simulink model "Planar_PIDC"  (R2022b)
settings: Solver=VariableStepAuto  StartTime=0.0  StopTime=40  RelTol=1e-3
values from neighbouring files (symbols this model uses):
  I = [1; 1; 1; 0.5; 0.5]*0.2    [RobDyn4link.m]
  l = [1; 1; 1; 1; 2]*0.2    [RobDyn4link.m]
  lc = l./2    [RobDyn4link.m]
  m = [1; 1; 1; 0.3; 0.3]*1    [RobDyn4link.m]
  q0 = [pi/2; -pi/4; -1*pi/6;-pi/12;0;]    [RobDyn4link.m]
  theta_max = [0.915*pi; 0.915*pi; 0.915*pi; 0.915*pi; 0.915*pi;]    [RobDyn4link.m]
  theta_min = [-0.915*pi; -0.915*pi; -0.915*pi; -0.915*pi; -0.915*pi;]    [RobDyn4link.m]
undefined symbols (not defined in the file or in its folder): DiscIntNeverNeededParam
(part 2 of 3)

== matlab function Planar_PIDC/Subsystem6/Subsystem1/MATLAB Function ==
  data: theta input; C output; dtheta input; m input; l input; lc input
function C = fcn(theta,dtheta,m,l,lc)
theta1 = theta(1); theta2 = theta(2); theta3 = theta(3); theta4 = theta(4); theta5 = theta(5);
dtheta1 = dtheta(1); dtheta2 = dtheta(2); dtheta3 = dtheta(3); dtheta4 = dtheta(4); dtheta5 = dtheta(5);
% I1 = I(1); I2 = I(2); I3 = I(3); I4 = I(4); I5 = I(5);
m1 = m(1); m2 = m(2); m3 = m(3); m4 = m(4); m5 = m(5);
l1 = l(1); l2 = l(2); l3 = l(3); l4 = l(4); l5 = l(5);
lc1 = lc(1); lc2 = lc(2); lc3 = lc(3); lc4 = lc(4); lc5 = lc(5);

 
C =[- dtheta2*l1*l4*m5*sin(theta2 + theta3 + theta4) - dtheta3*l1*l4*m5*sin(theta2 + theta3 + theta4) - dtheta4*l1*l4*m5*sin(theta2 + theta3 + theta4) - dtheta2*l1*lc4*m4*sin(theta2 + theta3 + theta4) - dtheta3*l1*lc4*m4*sin(theta2 + theta3 + theta4) - dtheta4*l1*lc4*m4*sin(theta2 + theta3 + theta4) - dtheta3*l2*lc5*m5*sin(theta3 + theta4 + theta5) - dtheta4*l2*lc5*m5*sin(theta3 + theta4 + theta5) - dtheta5*l2*lc5*m5*sin(theta3 + theta4 + theta5) - dtheta2*l1*lc5*m5*sin(theta2 + theta3 + theta4 + theta5) - dtheta3*l1*lc5*m5*sin(theta2 + theta3 + theta4 + theta5) - dtheta4*l1*lc5*m5*sin(theta2 + theta3 + theta4 + theta5) - dtheta5*l1*lc5*m5*sin(theta2 + theta3 + theta4 + theta5) - dtheta2*l1*l3*m4*sin(theta2 + theta3) - dtheta2*l1*l3*m5*sin(theta2 + theta3) - dtheta3*l1*l3*m4*sin(theta2 + theta3) - dtheta3*l1*l3*m5*sin(theta2 + theta3) - dtheta3*l2*l4*m5*sin(theta3 + theta4) - dtheta4*l2*l4*m5*sin(theta3 + theta4) - dtheta2*l1*lc3*m3*sin(theta2 + theta3) - dtheta3*l1*lc3*m3*sin(theta2 + theta3) - dtheta3*l2*lc4*m4*sin(theta3 + theta4) - dtheta4*l2*lc4*m4*sin(theta3 + theta4) - dtheta4*l3*lc5*m5*sin(theta4 + theta5) - dtheta5*l3*lc5*m5*sin(theta4 + theta5) - dtheta2*l1*l2*m3*sin(theta2) - dtheta2*l1*l2*m4*sin(theta2) - dtheta2*l1*l2*m5*sin(theta2) - dtheta3*l2*l3*m4*sin(theta3) - dtheta3*l2*l3*m5*sin(theta3) - dtheta4*l3*l4*m5*sin(theta4) - dtheta2*l1*lc2*m2*sin(theta2) - dtheta3*l2*lc3*m3*sin(theta3) - dtheta4*l3*lc4*m4*sin(theta4) - dtheta5*l4*lc5*m5*sin(theta5), - dtheta1*l1*l4*m5*sin(theta2 + theta3 + theta4) - dtheta2*l1*l4*m5*sin(theta2 + theta3 + theta4) - dtheta3*l1*l4*m5*sin(theta2 + theta3 + theta4) - dtheta4*l1*l4*m5*sin(theta2 + theta3 + theta4) - dtheta1*l1*lc4*m4*sin(theta2 + theta3 + theta4) - dtheta2*l1*lc4*m4*sin(theta2 + theta3 + theta4) - dtheta3*l1*lc4*m4*sin(theta2 + theta3 + theta4) - dtheta4*l1*lc4*m4*sin(theta2 + theta3 + theta4) - dtheta3*l2*lc5*m5*sin(theta3 + theta4 + theta5) - dtheta4*l2*lc5*m5*sin(theta3 + theta4 + theta5) - dtheta5*l2*lc5*m5*sin(theta3 + theta4 + theta5) - dtheta1*l1*lc5*m5*sin(theta2 + theta3 + theta4 + theta5) - dtheta2*l1*lc5*m5*sin(theta2 + theta3 + theta4 + theta5) - dtheta3*l1*lc5*m5*sin(theta2 + theta3 + theta4 + theta5) - dtheta4*l1*lc5*m5*sin(theta2 + theta3 + theta4 + theta5) - dtheta5*l1*lc5*m5*sin(theta2 + theta3 + theta4 + theta5) - dtheta1*l1*l3*m4*sin(theta2 + theta3) - dtheta1*l1*l3*m5*sin(theta2 + theta3) - dtheta2*l1*l3*m4*sin(theta2 + theta3) - dtheta2*l1*l3*m5*sin(theta2 + theta3) - dtheta3*l1*l3*m4*sin(theta2 + theta3) - dtheta3*l1*l3*m5*sin(theta2 + theta3) - dtheta3*l2*l4*m5*sin(theta3 + theta4) - dtheta4*l2*l4*m5*sin(theta3 + theta4) - dtheta1*l1*lc3*m3*sin(theta2 + theta3) - dtheta2*l1*lc3*m3*sin(theta2 + theta3) - dtheta3*l1*lc3*m3*sin(theta2 + theta3) - dtheta3*l2*lc4*m4*sin(theta3 + theta4) - dtheta4*l2*lc4*m4*sin(theta3 + theta4) - dtheta4*l3*lc5*m5*sin(theta4 + theta5) - dtheta5*l3*lc5*m5*sin(theta4 + theta5) - dtheta1*l1*l2*m3*sin(theta2) - dtheta1*l1*l2*m4*sin(theta2) - dtheta2*l1*l2*m3*sin(theta2) - dtheta1*l1*l2*m5*sin(theta2) - dtheta2*l1*l2*m4*sin(theta2) - dtheta2*l1*l2*m5*sin(theta2) - dtheta3*l2*l3*m4*sin(theta3) - dtheta3*l2*l3*m5*sin(theta3) - dtheta4*l3*l4*m5*sin(theta4) - dtheta1*l1*lc2*m2*sin(theta2) - dtheta2*l1*lc2*m2*sin(theta2) - dtheta3*l2*lc3*m3*sin(theta3) - dtheta4*l3*lc4*m4*sin(theta4) - dtheta5*l4*lc5*m5*sin(theta5), - dtheta1*l1*l4*m5*sin(theta2 + theta3 + theta4) - dtheta2*l1*l4*m5*sin(theta2 + theta3 + theta4) - dtheta3*l1*l4*m5*sin(theta2 + theta3 + theta4) - dtheta4*l1*l4*m5*sin(theta2 + theta3 + theta4) - dtheta1*l1*lc4*m4*sin(theta2 + theta3 + theta4) - dtheta2*l1*lc4*m4*sin(theta2 + theta3 + theta4) - dtheta3*l1*lc4*m4*sin(theta2 + theta3 + theta4) - dtheta4*l1*lc4*m4*sin(theta2 + theta3 + theta4) - dtheta1*l2*lc5*m5*sin(theta3 + theta4 + theta5) - dtheta2*l2*lc5*m5*sin(theta3 + theta4 + theta5) - dtheta3*l2*lc5*m5*sin(theta3 + theta4 + theta5) - dtheta4*l2*lc5*m5*sin(theta3 + theta4 + theta5) - dtheta5*l2*lc5*m5*sin(theta3 + theta4 + theta5) - dtheta1*l1*lc5*m5*sin(theta2 + theta3 + theta4 + theta5) - dtheta2*l1*lc5*m5*sin(theta2 + theta3 + theta4 + theta5) - dtheta3*l1*lc5*m5*sin(theta2 + theta3 + theta4 + theta5) - dtheta4*l1*lc5*m5*sin(theta2 + theta3 + theta4 + theta5) - dtheta5*l1*lc5*m5*sin(theta2 + theta3 + theta4 + theta5) - dtheta1*l1*l3*m4*sin(theta2 + theta3) - dtheta1*l1*l3*m5*sin(theta2 + theta3) - dtheta2*l1*l3*m4*sin(theta2 + theta3) - dtheta2*l1*l3*m5*sin(theta2 + theta3) - dtheta3*l1*l3*m4*sin(theta2 + theta3) - dtheta3*l1*l3*m5*sin(theta2 + theta3) - dtheta1*l2*l4*m5*sin(theta3 + theta4) - dtheta2*l2*l4*m5*sin(theta3 + theta4) - dtheta3*l2*l4*m5*sin(theta3 + theta4) - dtheta4*l2*l4*m5*sin(theta3 + theta4) - dtheta1*l1*lc3*m3*sin(theta2 + theta3) - dtheta2*l1*lc3*m3*sin(theta2 + theta3) - dtheta3*l1*lc3*m3*sin(theta2 + theta3) - dtheta1*l2*lc4*m4*sin(theta3 + theta4) - dtheta2*l2*lc4*m4*sin(theta3 + theta4) - dtheta3*l2*lc4*m4*sin(theta3 + theta4) - dtheta4*l2*lc4*m4*sin(theta3 + theta4) - dtheta4*l3*lc5*m5*sin(theta4 + theta5) - dtheta5*l3*lc5*m5*sin(theta4 + theta5) - dtheta1*l2*l3*m4*sin(theta3) - dtheta1*l2*l3*m5*sin(theta3) - dtheta2*l2*l3*m4*sin(theta3) - dtheta2*l2*l3*m5*sin(theta3) - dtheta3*l2*l3*m4*sin(theta3) - dtheta3*l2*l3*m5*sin(theta3) - dtheta4*l3*l4*m5*sin(theta4) - dtheta1*l2*lc3*m3*sin(theta3) - dtheta2*l2*lc3*m3*sin(theta3) - dtheta3*l2*lc3*m3*sin(theta3) - dtheta4*l3*lc4*m4*sin(theta4) - dtheta5*l4*lc5*m5*sin(theta5), - dtheta1*l1*l4*m5*sin(theta2 + theta3 + theta4) - dtheta2*l1*l4*m5*sin(theta2 + theta3 + theta4) - dtheta3*l1*l4*m5*sin(theta2 + theta3 + theta4) - dtheta4*l1*l4*m5*sin(theta2 + theta3 + theta4) - dtheta1*l1*lc4*m4*sin(theta2 + theta3 + theta4) - dtheta2*l1*lc4*m4*sin(theta2 + theta3 + theta4) - dtheta3*l1*lc4*m4*sin(theta2 + theta3 + theta4) - dtheta4*l1*lc4*m4*sin(theta2 + theta3 + theta4) - dtheta1*l2*lc5*m5*sin(theta3 + theta4 + theta5) - dtheta2*l2*lc5*m5*sin(theta3 + theta4 + theta5) - dtheta3*l2*lc5*m5*sin(theta3 + theta4 + theta5) - dtheta4*l2*lc5*m5*sin(theta3 + theta4 + theta5) - dtheta5*l2*lc5*m5*sin(theta3 + theta4 + theta5) - dtheta1*l1*lc5*m5*sin(theta2 + theta3 + theta4 + theta5) - dtheta2*l1*lc5*m5*sin(theta2 + theta3 + theta4 + theta5) - dtheta3*l1*lc5*m5*sin(theta2 + theta3 + theta4 + theta5) - dtheta4*l1*lc5*m5*sin(theta2 + theta3 + theta4 + theta5) - dtheta5*l1*lc5*m5*sin(theta2 + theta3 + theta4 + theta5) - dtheta1*l2*l4*m5*sin(theta3 + theta4) - dtheta2*l2*l4*m5*sin(theta3 + theta4) - dtheta3*l2*l4*m5*sin(theta3 + theta4) - dtheta4*l2*l4*m5*sin(theta3 + theta4) - dtheta1*l2*lc4*m4*sin(theta3 + theta4) - dtheta2*l2*lc4*m4*sin(theta3 + theta4) - dtheta3*l2*lc4*m4*sin(theta3 + theta4) - dtheta4*l2*lc4*m4*sin(theta3 + theta4) - dtheta1*l3*lc5*m5*sin(theta4 + theta5) - dtheta2*l3*lc5*m5*sin(theta4 + theta5) - dtheta3*l3*lc5*m5*sin(theta4 + theta5) - dtheta4*l3*lc5*m5*sin(theta4 + theta5) - dtheta5*l3*lc5*m5*sin(theta4 + theta5) - dtheta1*l3*l4*m5*sin(theta4) - dtheta2*l3*l4*m5*sin(theta4) - dtheta3*l3*l4*m5*sin(theta4) - dtheta4*l3*l4*m5*sin(theta4) - dtheta1*l3*lc4*m4*sin(theta4) - dtheta2*l3*lc4*m4*sin(theta4) - dtheta3*l3*lc4*m4*sin(theta4) - dtheta4*l3*lc4*m4*sin(theta4) - dtheta5*l4*lc5*m5*sin(theta5), -lc5*m5*(l1*sin(theta2 + theta3 + theta4 + theta5) + l3*sin(theta4 + theta5) + l4*sin(theta5) + l2*sin(theta3 + theta4 + theta5))*(dtheta1 + dtheta2 + dtheta3 + dtheta4 + dtheta5);
                                                                                                                                                                                                                                                                                                                                                                                                                                                                                                                  dtheta1*l1*l4*m5*sin(theta2 + theta3 + theta4) + dtheta1*l1*lc4*m4*sin(theta2 + theta3 + theta4) - dtheta3*l2*lc5*m5*sin(theta3 + theta4 + theta5) - dtheta4*l2*lc5*m5*sin(theta3 + theta4 + theta5) - dtheta5*l2*lc5*m5*sin(theta3 + theta4 + theta5) + dtheta1*l1*lc5*m5*sin(theta2 + theta3 + theta4 + theta5) + dtheta1*l1*l3*m4*sin(theta2 + theta3) + dtheta1*l1*l3*m5*sin(theta2 + theta3) - dtheta3*l2*l4*m5*sin(theta3 + theta4) - dtheta4*l2*l4*m5*sin(theta3 + theta4) + dtheta1*l1*lc3*m3*sin(theta2 + theta3) - dtheta3*l2*lc4*m4*sin(theta3 + theta4) - dtheta4*l2*lc4*m4*sin(theta3 + theta4) - dtheta4*l3*lc5*m5*sin(theta4 + theta5) - dtheta5*l3*lc5*m5*sin(theta4 + theta5) + dtheta1*l1*l2*m3*sin(theta2) + dtheta1*l1*l2*m4*sin(theta2) + dtheta1*l1*l2*m5*sin(theta2) - dtheta3*l2*l3*m4*sin(theta3) - dtheta3*l2*l3*m5*sin(theta3) - dtheta4*l3*l4*m5*sin(theta4) + dtheta1*l1*lc2*m2*sin(theta2) - dtheta3*l2*lc3*m3*sin(theta3) - dtheta4*l3*lc4*m4*sin(theta4) - dtheta5*l4*lc5*m5*sin(theta5),                                                                                                                                                                                                                                                                                                                                                                                                                                                                                                                                                                                                                                                                                                                                                                                                                                                                                                                                                                                                                                                                                                                                                                                                                                                                                                                                                                                                                                                                                - dtheta4*(l2*l4*m5*sin(theta3 + theta4) + l2*lc4*m4*sin(theta3 + theta4) + l3*lc5*m5*sin(theta4 + theta5) + l3*l4*m5*sin(theta4) + l3*lc4*m4*sin(theta4) + l2*lc5*m5*sin(theta3 + theta4 + theta5)) - dtheta3*l2*(l3*m4*sin(theta3) + l3*m5*sin(theta3) + lc3*m3*sin(theta3) + lc5*m5*sin(theta3 + theta4 + theta5) + l4*m5*sin(theta3 + theta4) + lc4*m4*sin(theta3 + theta4)) - dtheta5*lc5*m5*(l3*sin(theta4 + theta5) + l4*sin(theta5) + l2*sin(theta3 + theta4 + theta5)),                                                                                                                                                                                                                                                                                                                                                                                                                                                                                                                                                                                                                                                                                                                                                                                                                                                                                                                                                                                                                                                                                               - dtheta1*l2*lc5*m5*sin(theta3 + theta4 + theta5) - dtheta2*l2*lc5*m5*sin(theta3 + theta4 + theta5) - dtheta3*l2*lc5*m5*sin(theta3 + theta4 + theta5) - dtheta4*l2*lc5*m5*sin(theta3 + theta4 + theta5) - dtheta5*l2*lc5*m5*sin(theta3 + theta4 + theta5) - dtheta1*l2*l4*m5*sin(theta3 + theta4) - dtheta2*l2*l4*m5*sin(theta3 + theta4) - dtheta3*l2*l4*m5*sin(theta3 + theta4) - dtheta4*l2*l4*m5*sin(theta3 + theta4) - dtheta1*l2*lc4*m4*sin(theta3 + theta4) - dtheta2*l2*lc4*m4*sin(theta3 + theta4) - dtheta3*l2*lc4*m4*sin(theta3 + theta4) - dtheta4*l2*lc4*m4*sin(theta3 + theta4) - dtheta4*l3*lc5*m5*sin(theta4 + theta5) - dtheta5*l3*lc5*m5*sin(theta4 + theta5) - dtheta1*l2*l3*m4*sin(theta3) - dtheta1*l2*l3*m5*sin(theta3) - dtheta2*l2*l3*m4*sin(theta3) - dtheta2*l2*l3*m5*sin(theta3) - dtheta3*l2*l3*m4*sin(theta3) - dtheta3*l2*l3*m5*sin(theta3) - dtheta4*l3*l4*m5*sin(theta4) - dtheta1*l2*lc3*m3*sin(theta3) - dtheta2*l2*lc3*m3*sin(theta3) - dtheta3*l2*lc3*m3*sin(theta3) - dtheta4*l3*lc4*m4*sin(theta4) - dtheta5*l4*lc5*m5*sin(theta5),                                                                                                                                                                                                                                                                                                                                                                                                                                                                                                                                                                                                                                                                                                                    - dtheta1*l2*lc5*m5*sin(theta3 + theta4 + theta5) - dtheta2*l2*lc5*m5*sin(theta3 + theta4 + theta5) - dtheta3*l2*lc5*m5*sin(theta3 + theta4 + theta5) - dtheta4*l2*lc5*m5*sin(theta3 + theta4 + theta5) - dtheta5*l2*lc5*m5*sin(theta3 + theta4 + theta5) - dtheta1*l2*l4*m5*sin(theta3 + theta4) - dtheta2*l2*l4*m5*sin(theta3 + theta4) - dtheta3*l2*l4*m5*sin(theta3 + theta4) - dtheta4*l2*l4*m5*sin(theta3 + theta4) - dtheta1*l2*lc4*m4*sin(theta3 + theta4) - dtheta2*l2*lc4*m4*sin(theta3 + theta4) - dtheta3*l2*lc4*m4*sin(theta3 + theta4) - dtheta4*l2*lc4*m4*sin(theta3 + theta4) - dtheta1*l3*lc5*m5*sin(theta4 + theta5) - dtheta2*l3*lc5*m5*sin(theta4 + theta5) - dtheta3*l3*lc5*m5*sin(theta4 + theta5) - dtheta4*l3*lc5*m5*sin(theta4 + theta5) - dtheta5*l3*lc5*m5*sin(theta4 + theta5) - dtheta1*l3*l4*m5*sin(theta4) - dtheta2*l3*l4*m5*sin(theta4) - dtheta3*l3*l4*m5*sin(theta4) - dtheta4*l3*l4*m5*sin(theta4) - dtheta1*l3*lc4*m4*sin(theta4) - dtheta2*l3*lc4*m4*sin(theta4) - dtheta3*l3*lc4*m4*sin(theta4) - dtheta4*l3*lc4*m4*sin(theta4) - dtheta5*l4*lc5*m5*sin(theta5),                                             -lc5*m5*(l3*sin(theta4 + theta5) + l4*sin(theta5) + l2*sin(theta3 + theta4 + theta5))*(dtheta1 + dtheta2 + dtheta3 + dtheta4 + dtheta5);
                                                                                                                                                                                                                                                                                                                                                                                                                                                                                                                                                                                                   dtheta1*l1*l4*m5*sin(theta2 + theta3 + theta4) + dtheta1*l1*lc4*m4*sin(theta2 + theta3 + theta4) + dtheta1*l2*lc5*m5*sin(theta3 + theta4 + theta5) + dtheta2*l2*lc5*m5*sin(theta3 + theta4 + theta5) + dtheta1*l1*lc5*m5*sin(theta2 + theta3 + theta4 + theta5) + dtheta1*l1*l3*m4*sin(theta2 + theta3) + dtheta1*l1*l3*m5*sin(theta2 + theta3) + dtheta1*l2*l4*m5*sin(theta3 + theta4) + dtheta2*l2*l4*m5*sin(theta3 + theta4) + dtheta1*l1*lc3*m3*sin(theta2 + theta3) + dtheta1*l2*lc4*m4*sin(theta3 + theta4) + dtheta2*l2*lc4*m4*sin(theta3 + theta4) - dtheta4*l3*lc5*m5*sin(theta4 + theta5) - dtheta5*l3*lc5*m5*sin(theta4 + theta5) + dtheta1*l2*l3*m4*sin(theta3) + dtheta1*l2*l3*m5*sin(theta3) + dtheta2*l2*l3*m4*sin(theta3) + dtheta2*l2*l3*m5*sin(theta3) - dtheta4*l3*l4*m5*sin(theta4) + dtheta1*l2*lc3*m3*sin(theta3) + dtheta2*l2*lc3*m3*sin(theta3) - dtheta4*l3*lc4*m4*sin(theta4) - dtheta5*l4*lc5*m5*sin(theta5),                                                                                                                                                                                                                                                                                                                                                                                                                                                                                                                                                                                                                                                                                                                                                                                                                                                                                                                                                                                                                                                                                                                                                                                                                                                                                                                                                                                                               dtheta1*(l2*l4*m5*sin(theta3 + theta4) + l2*lc4*m4*sin(theta3 + theta4) + l2*l3*m4*sin(theta3) + l2*l3*m5*sin(theta3) + l2*lc3*m3*sin(theta3) + l2*lc5*m5*sin(theta3 + theta4 + theta5)) - dtheta5*(l3*lc5*m5*sin(theta4 + theta5) + l4*lc5*m5*sin(theta5)) + dtheta2*(l2*l4*m5*sin(theta3 + theta4) + l2*lc4*m4*sin(theta3 + theta4) + l2*l3*m4*sin(theta3) + l2*l3*m5*sin(theta3) + l2*lc3*m3*sin(theta3) + l2*lc5*m5*sin(theta3 + theta4 + theta5)) - dtheta4*(l3*lc5*m5*sin(theta4 + theta5) + l3*l4*m5*sin(theta4) + l3*lc4*m4*sin(theta4)),                                                                                                                                                                                                                                                                                                                                                                                                                                                                                                                                                                                                                                                                                                                                                                                                                                                                                                                                                                                                                                                                                                                                                                                                                                                                                                                                                                                                                                                                                                                                                                                                                                                                                                                                                                                                                                                                                                                                                                                                           - dtheta5*(l3*lc5*m5*sin(theta4 + theta5) + l4*lc5*m5*sin(theta5)) - dtheta4*(l3*lc5*m5*sin(theta4 + theta5) + l3*l4*m5*sin(theta4) + l3*lc4*m4*sin(theta4)),                                                                                                                                                                                                                                                                                                                                                                                                                                                                                                                                                                                                                                                                                                                                                                                                                                                                                                                                                                                                                                                                                                                                                                                                                                                                                                                                                                                                               - dtheta1*l3*(l4*m5*sin(theta4) + lc4*m4*sin(theta4) + lc5*m5*sin(theta4 + theta5)) - dtheta2*l3*(l4*m5*sin(theta4) + lc4*m4*sin(theta4) + lc5*m5*sin(theta4 + theta5)) - dtheta3*l3*(l4*m5*sin(theta4) + lc4*m4*sin(theta4) + lc5*m5*sin(theta4 + theta5)) - dtheta4*l3*(l4*m5*sin(theta4) + lc4*m4*sin(theta4) + lc5*m5*sin(theta4 + theta5)) - dtheta5*lc5*m5*(l3*sin(theta4 + theta5) + l4*sin(theta5)),                                                                                -lc5*m5*(l3*sin(theta4 + theta5) + l4*sin(theta5))*(dtheta1 + dtheta2 + dtheta3 + dtheta4 + dtheta5);
                                                                                                                                                                                                                                                                                                                                                                                                                                                                                                                                                                                                                                                                                                                                                 dtheta1*l1*l4*m5*sin(theta2 + theta3 + theta4) + dtheta1*l1*lc4*m4*sin(theta2 + theta3 + theta4) + dtheta1*l2*lc5*m5*sin(theta3 + theta4 + theta5) + dtheta2*l2*lc5*m5*sin(theta3 + theta4 + theta5) + dtheta1*l1*lc5*m5*sin(theta2 + theta3 + theta4 + theta5) + dtheta1*l2*l4*m5*sin(theta3 + theta4) + dtheta2*l2*l4*m5*sin(theta3 + theta4) + dtheta1*l2*lc4*m4*sin(theta3 + theta4) + dtheta2*l2*lc4*m4*sin(theta3 + theta4) + dtheta1*l3*lc5*m5*sin(theta4 + theta5) + dtheta2*l3*lc5*m5*sin(theta4 + theta5) + dtheta3*l3*lc5*m5*sin(theta4 + theta5) + dtheta1*l3*l4*m5*sin(theta4) + dtheta2*l3*l4*m5*sin(theta4) + dtheta3*l3*l4*m5*sin(theta4) + dtheta1*l3*lc4*m4*sin(theta4) + dtheta2*l3*lc4*m4*sin(theta4) + dtheta3*l3*lc4*m4*sin(theta4) - dtheta5*l4*lc5*m5*sin(theta5),                                                                                                                                                                                                                                                                                                                                                                                                                                                                                                                                                                                                                                                                                                                                                                                                                                                                                                                                                                                                                                                                                                                                                                                                                                                                                                                                    dtheta1*l2*lc5*m5*sin(theta3 + theta4 + theta5) + dtheta2*l2*lc5*m5*sin(theta3 + theta4 + theta5) + dtheta1*l2*l4*m5*sin(theta3 + theta4) + dtheta2*l2*l4*m5*sin(theta3 + theta4) + dtheta1*l2*lc4*m4*sin(theta3 + theta4) + dtheta2*l2*lc4*m4*sin(theta3 + theta4) + dtheta1*l3*lc5*m5*sin(theta4 + theta5) + dtheta2*l3*lc5*m5*sin(theta4 + theta5) + dtheta3*l3*lc5*m5*sin(theta4 + theta5) + dtheta1*l3*l4*m5*sin(theta4) + dtheta2*l3*l4*m5*sin(theta4) + dtheta3*l3*l4*m5*sin(theta4) + dtheta1*l3*lc4*m4*sin(theta4) + dtheta2*l3*lc4*m4*sin(theta4) + dtheta3*l3*lc4*m4*sin(theta4) - dtheta5*l4*lc5*m5*sin(theta5),                                                                                                                                                                                                                                                                                                                                                                                                                                                                                                                                                                                                                                                                                                                                                                                                                                                                                                                                                                                                                                                                                                                                                                                                                                                                                                                                                                                                                                                                                                                                                                                                                                                                                                                                                                                                                                                                              dtheta1*l3*(l4*m5*sin(theta4) + lc4*m4*sin(theta4) + lc5*m5*sin(theta4 + theta5)) + dtheta2*l3*(l4*m5*sin(theta4) + lc4*m4*sin(theta4) + lc5*m5*sin(theta4 + theta5)) + dtheta3*l3*(l4*m5*sin(theta4) + lc4*m4*sin(theta4) + lc5*m5*sin(theta4 + theta5)) - dtheta5*l4*lc5*m5*sin(theta5),                                                                                                                                                                                                                                                                                                                                                                                                                                                                                                                                                                                                                                                                                                                                                                                                                                                                                                                                                                                                                                                                                                                                                                                                                                                                                                                                                                                                                                                                                                                                                                                                                                                                                                                                                                                            -dtheta5*l4*lc5*m5*sin(theta5),                                                                                                            -l4*lc5*m5*sin(theta5)*(dtheta1 + dtheta2 + dtheta3 + dtheta4 + dtheta5);
                                                                                                                                                                                                                                                                                                                                                                                                                                                                                                                                                                                                                                                                                                                                                                                                                                                                                                                                                                                                                                                                                                                                                                                lc5*m5*(dtheta1*l4*sin(theta5) + dtheta2*l4*sin(theta5) + dtheta3*l4*sin(theta5) + dtheta4*l4*sin(theta5) + dtheta1*l2*sin(theta3 + theta4 + theta5) + dtheta2*l2*sin(theta3 + theta4 + theta5) + dtheta1*l1*sin(theta2 + theta3 + theta4 + theta5) + dtheta1*l3*sin(theta4 + theta5) + dtheta2*l3*sin(theta4 + theta5) + dtheta3*l3*sin(theta4 + theta5)),                                                                                                                                                                                                                                                                                                                                                                                                                                                                                                                                                                                                                                                                                                                                                                                                                                                                                                                                                                                                                                                                                                                                                                                                                                                                                                                                                                                                                                                                                                                                                                                                                                                         lc5*m5*(dtheta1*l4*sin(theta5) + dtheta2*l4*sin(theta5) + dtheta3*l4*sin(theta5) + dtheta4*l4*sin(theta5) + dtheta1*l2*sin(theta3 + theta4 + theta5) + dtheta2*l2*sin(theta3 + theta4 + theta5) + dtheta1*l3*sin(theta4 + theta5) + dtheta2*l3*sin(theta4 + theta5) + dtheta3*l3*sin(theta4 + theta5)),                                                                                                                                                                                                                                                                                                                                                                                                                                                                                                                                                                                                                                                                                                                                                                                                                                                                                                                                                                                                                                                                                                                                                                                                                                                                                                                                                                                                                                                                                                                                                                                                                                                                                                                                                                                                                                                                                                                                                       lc5*m5*(dtheta1*l4*sin(theta5) + dtheta2*l4*sin(theta5) + dtheta3*l4*sin(theta5) + dtheta4*l4*sin(theta5) + dtheta1*l3*sin(theta4 + theta5) + dtheta2*l3*sin(theta4 + theta5) + dtheta3*l3*sin(theta4 + theta5)),                                                                                                                                                                                                                                                                                                                                                                                                                                                                                                                                                                                                                                                                                                                                                                                                                                                                                                                                                                                                                                                                                                                                                                                                                                                                                                                                                                                                                                                                                                                                                                                                                                                                                                                                                             l4*lc5*m5*sin(theta5)*(dtheta1 + dtheta2 + dtheta3 + dtheta4),                                                                                                                                                                                   0;];

== matlab function Planar_PIDC/Subsystem1/MATLAB Function1 ==
  data: xdot input; y output; x input; xd input; xd_dot input
function y = fcn(xdot,x, xd, xd_dot)

m = 5;
Kp = 10;
% xd = 1;
y = 0.5*m*(xdot - xd_dot)^2 + 0.5*Kp*(x - xd)^2;

== matlab function Planar_PIDC/Subsystem3/Subsystem2/MATLAB Function5 ==
  data: Lambda_c output size=[3,3]; Hc output; J_general input; J_generaldot input; Jee input; Jeedot input; M input; C input; thetadot input; Mbar output; P output
function [Lambda_c,Hc,Mbar,P] = fcn(J_general,J_generaldot,Jee,Jeedot,M,C,thetadot)
Jc = J_general;
Jc_pinv = Jc'/(Jc*Jc' + 0*eye(1));
P = eye(5) - Jc_pinv*Jc;

%% previous part
Pnull = eye(5) - P;
Mc = P*M + (eye(5) - P);
% Lambda_c = (Jee * (Mc \ P) * Jee'+ 1e-3*eye(3) ) \ eye(3);
% 
% PMP = P*M*P;
% McInvP = PMP'*(PMP*PMP');
% % Lambda_c = eye(3)/(Jee*McInvP*Jee'+1e-1*eye(3));
% 
% coder.extrinsic('computeLambdaC');
% Lambda_c = eye(3);
% Lambda_c = computeLambdaC(Jee,Mc,P,1e-6);

%% Farhad Aghili 2016 ICRA
nv = 0.5;
Mbar = P*M*P + nv*(eye(5) - P);
S = eye(5) - M/Mbar*P;
Jcdot = J_generaldot;
Gamma = -Jc_pinv*Jcdot;
Omega = Gamma - Gamma';

coder.extrinsic('svdInverse');
Lambda_c = eye(3);
Lambda_c = svdInverse(Jee*(Mbar \ P)*Jee',1e-4);
% Lambda_c = (Jee*(Mbar \ P)*Jee' + 1e-2*eye(3)) \ eye(3);

Hc = Lambda_c*(Jee/Mbar*(Mbar*S'*Omega*thetadot + P*C*thetadot) - Jeedot*thetadot);

== matlab function Planar_PIDC/Subsystem1/MATLAB Function2 ==
  data: xd_ddot input; xd_dot input; edot input; y output; e input
function y = fcn(xd_ddot,xd_dot, edot, e)
M = 5;
D = 1;
Kp = 10;
% Kd = sqrt(Kp/M)*2;
Kd = 2;
y = 1*M*xd_ddot + 1*D*xd_dot + Kd*edot + Kp*e;

== matlab function Planar_PIDC/Subsystem1/MATLAB Function3 ==
  data: t input; y output; yd output; ydd output
function [y,yd,ydd]= fcn(t)

y = sin(t);
yd = cos(t);
ydd = -sin(t);

== matlab function Planar_PIDC/Subsystem3/MATLAB Function5 ==
  data: u input; y output
function y = fcn(u)

y = norm(u);
